simulink model "aero_control"  (Simulink 7.5)
settings: Solver=ode45  StartTime=0.0  StopTime=10.0  RelTol=1e-3
values from neighbouring files (symbols this model uses):
  CL1 = (1/2)*DiffCLZeta*Sf*Nf*Lf3    (= 2.0002634928)    [valuables.m]
  CM4 = (-1/2)*DiffCLZeta*Sf*Nf*Lf1    (= -12.84322188)    [valuables.m]
  CY4 = (-1/2)*DiffCLZeta*Sf*Nf    (= -1.8217336)    [valuables.m]
settings Model: Creator=ex08148  LastModifiedBy=ex08148

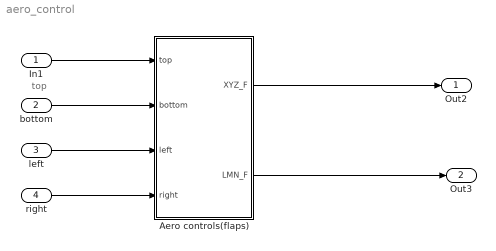
== system aero_control ==
  note: top
  In1 : Inport  OutDataType=sfix(16)  OutScaling=2^0
  bottom : Inport  Port=2  OutDataType=sfix(16)  OutScaling=2^0
  left : Inport  Port=3  OutDataType=sfix(16)  OutScaling=2^0
  right : Inport  Port=4  OutDataType=sfix(16)  OutScaling=2^0
  Aero controls(flaps) : Subsystem
  "Out2 " : Outport  OutDataType=sfix(16)  OutScaling=2^0
  Out3 : Outport  Port=2  OutDataType=sfix(16)  OutScaling=2^0
  wires:
  Aero controls(flaps)/1(XYZ_F) -> "Out2 "/1
  Aero controls(flaps)/2(LMN_F) -> Out3/1
  In1/1 -> Aero controls(flaps)/1(top)
  bottom/1 -> Aero controls(flaps)/2(bottom)
  left/1 -> Aero controls(flaps)/3(left)
  right/1 -> Aero controls(flaps)/4(right)

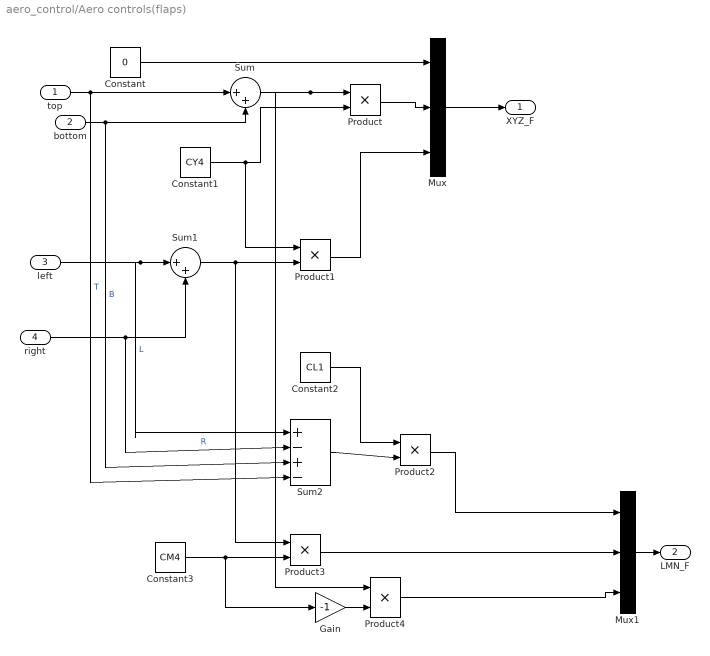
== system aero_control/Aero controls(flaps) ==
  top : Inport  OutDataType=sfix(16)  OutScaling=2^0
  bottom : Inport  Port=2  OutDataType=sfix(16)  OutScaling=2^0
  left : Inport  Port=3  OutDataType=sfix(16)  OutScaling=2^0
  right : Inport  Port=4  OutDataType=sfix(16)  OutScaling=2^0
  Constant : Constant  Value=0  OutDataType=sfix(16)  OutScaling=2^0
  Constant1 : Constant  Value=CY4  OutDataType=sfix(16)  OutScaling=2^0
  Constant2 : Constant  Value=CL1  OutDataType=sfix(16)  OutScaling=2^0
  Constant3 : Constant  Value=CM4  OutDataType=sfix(16)  OutScaling=2^0
  Gain : Gain  Gain=-1  ParameterDataType=sfix(16)  ParameterScaling=2^0  OutDataType=sfix(16)  OutScaling=2^0
  Mux : Mux  Inputs=3
  Mux1 : Mux  Inputs=3
  Product{,1..4} (5 alike) : Product  OutDataType=sfix(16)  OutScaling=2^0  RndMeth=Zero
  Sum : Sum  Inputs=|++  OutDataType=sfix(16)  OutScaling=2^0
  Sum1 : Sum  Inputs=|++  OutDataType=sfix(16)  OutScaling=2^0
  Sum2 : Sum  Inputs=|+-+-  OutDataType=sfix(16)  OutScaling=2^0
  XYZ_F : Outport  OutDataType=sfix(16)  OutScaling=2^0
  LMN_F : Outport  Port=2  OutDataType=sfix(16)  OutScaling=2^0
  wires:
  top/1 -> Sum/1, Sum2/4  "T"
  bottom/1 -> Sum/2, Sum2/3  "B"
  Sum/1 -> Product/1, Product4/1
  Constant1/1 -> Product/2, Product1/1
  left/1 -> Sum1/1, Sum2/1  "L"
  right/1 -> Sum1/2, Sum2/2  "R"
  Sum1/1 -> Product1/2, Product3/1
  Constant/1 -> Mux/1
  Product/1 -> Mux/2
  Product1/1 -> Mux/3
  Sum2/1 -> Product2/2
  Constant2/1 -> Product2/1
  Constant3/1 -> Product3/2, Gain/1
  Product4/1 -> Mux1/3
  Product3/1 -> Mux1/2
  Product2/1 -> Mux1/1
  Mux/1 -> XYZ_F/1
  Mux1/1 -> LMN_F/1
  Gain/1 -> Product4/2
